simulink model "PistonController3"  (R2013a)
settings: Solver=FixedStepDiscrete  StartTime=0.0  StopTime=30  FixedStep=0.001  RelTol=1e-3
InitFcn:
  | % PI gains
  | 
  | K1_crit = 17.0;
  | T1_crit = 1.75;
  | K2_crit = K1_crit;
  | T2_crit = T1_crit;
  | K3_crit = K1_crit;
  | T3_crit = T1_crit;
  | K4_crit = K1_crit;
  | T4_crit = T1_crit;
  | K5_crit = 5.0;
  | T5_crit = 0.5;
  | K6_crit = 17.0;
  | T6_crit = 1.75;
  | KG_crit = 10.0;
  | TG_crit = 1.75;
  | 
  | 
  | P1 = 0.2*K1_crit;
  | I1 = 3.0*P1/T1_crit;
  | D1 = P1*T1_crit/3.0;
  | N1 = 10.0;
  | 
  | P2 = 0.2*K2_crit;
  | I2 = 3.0*P2/T2_crit;
  | D2 = P2*T2_crit/3.0;
  | N2 = 10.0;
  | 
  | P3 = 0.2*K3_crit;
  | I3 = 3.0*P3/T3_crit;
  | D3 = P3*T3_crit/3.0;
  | N3 = 10.0;
  | 
  | P4 = 0.2*K4_crit;
  | I4 = 3.0*P4/T4_crit;
  | D4 = P4*T4_crit/3.0;
  | N4 = 10.0;
  | 
  | P5 = 0.45*K5_crit;
  | I5 = 1.2*P5/T5_crit;
  | D5 = 0; %P5*T5_crit/3.0;
  | N5 = 10.0;
  | 
  | P6 = 0.2*K6_crit;
  | I6 = 3.0*P6/T6_crit;
  | D6 = P6*T6_crit/3.0;
  | N6 = 10.0;
  | 
  | PG = 0.2*KG_crit;
  | IG = 3.0*PG/TG_crit;
  | DG = PG*TG_crit/3.0;
  | NG = 10.0;
  | 
  | % offsets
  | offset = 1000;
  | offset_grip = 0;
  | 
  | %Max Cylinder Displacements = Left = positive
  | max_pos1 = 2800;
  | min_pos1 = -2800;
  | 
  | max_pos2 = 3000;
  | min_pos2 = -2700;
  | 
  | max_pos3 = 3000;
  | min_pos3 = -3000;
  | 
  | max_pos4 = 2800;
  | min_pos4 = -2900;
  | 
  | max_pos5 = 2900;
  | min_pos5 = -2600;
  | 
  | max_pos6 = 2800;
  | min_pos6 = -2800;
  | 
  | max_posG = 1500;
  | 
  | %Max Control Efforts
  | max1 = 5600;
  | min1 = -5600;
  | 
  | max2 = 5700;
  | min2 = -5700;
  | 
  | max3 = 6000;
  | min3 = -6000;
  | 
  | max4 = 5700;
  | min4 = -5700;
  | 
  | max5 = 5500;
  | min5 = -5500;
  | 
  | max6 = 5600;
  | min6 = -5600;
  | 
  | maxG = 3000;
  | minG = -3000;
undefined symbols (not defined in the file): rtwindemocb_modeswitch, Serial_Port, Standard_Devices
libraries: rtwinlib x14, simulink x7
Description:
  | Packet Input/Output
  | 
  | This model shows how to transfer data through UDP
  | communication protocol using binary encoding. The model sends data
  | within one computer, from one UDP port to another. You can modify the
  | model to communicate between two computers by splitting this model
  | into its send and receive parts and running the models on two computers.
  | The yellow blocks are used to send the data, the blue blocks
  | are used to receive the data. Then, please enter the IP addresses of the two
  | computers into the appropriate fields in the Board Setup dialog.
  | 
  | How to run this model in Normal Mode:
  | 
  | 1) Double-click the orange button to switch to Normal Mode if needed.
  | 2) Start the real-time execution using Simulation->Run.
  | 
  | How to run this model in External Mode:
  | 
  | 1) Double-click the orange button to switch to External Mode if needed.
  | 2) Build the model using Code->C/C++ Code->Build Model.
  | 3) Connect to the real-time code using Simulation->Connect To Target.
  | 4) Start the real-time execution using Simulation->Run.
settings Model: SimulationMode=external  ExtModeTrigDuration=30001  Creator=The MathWorks Inc.  LastModifiedBy=drl
settings DataIOCC: SignalLoggingSaveFormat=ModelDataLogs
settings OptimizationCC: InlineParams=on  InlineInvariantSignals=on  EnhancedBackFolding=on  ExpressionDepthLimit=2147483647  InitFltsAndDblsToZero=on  EfficientFloat2IntCast=on  EfficientMapNaN2IntZero=off  SimCompilerOptimization=On
settings DebuggingCC: MultiTaskDSMMsg=warning  MultiTaskCondExecSysMsg=none  FcnCallInpInsideContextMsg=EnableAllAsWarning  StrictBusMsg=None
settings HardwareCC: ProdIntDivRoundTo=Zero  ProdEndianess=LittleEndian  ProdHWDeviceType=32-bit Real-Time Windows Target  TargetIntDivRoundTo=Zero  TargetEndianess=LittleEndian  TargetHWDeviceType=32-bit Real-Time Windows Target
settings ModelReferenceCC: UpdateModelReferenceTargets=IfOutOfDate
settings SFSimCC: SFSimEcho=off
settings RTWCC: SystemTargetFile=rtwin.tlc  TemplateMakefile=rtwin.tmf  Description=Real-Time Windows Target  ProcessScript=rtwin_make_rtw_hook  IncludeERTFirstTime=on  RTWCompilerOptimization=On
settings RTWinTargetCC: TargetLibSuffix=_rtwin.lib  TargetPreCompLibLocation=C:\Program Files\MATLAB\R2013a\toolbox\rtw\targets\rtwin\lib\win64  CodeReplacementLibrary=ANSI_C  RTWinDir=C:/PROGRA~1/MATLAB/R2013a/toolbox/rtw/targets/rtwin  TargetArch=win64

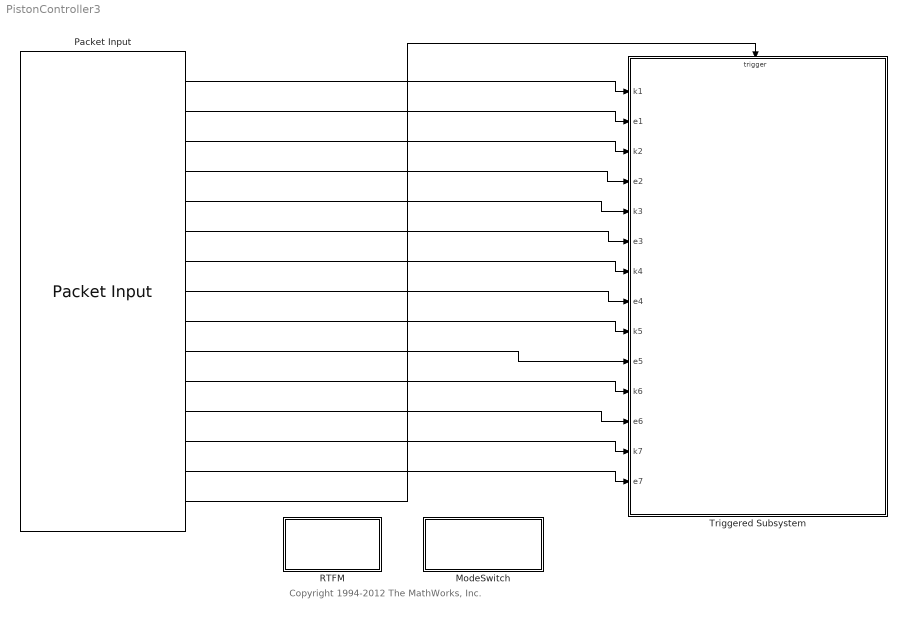
== system PistonController3 ==
  note: Copyright 1994-2012 The MathWorks, Inc.
  ModeSwitch : Subsystem  InitFcn=rtwindemocb_modeswitch('CheckKernel');  mask(Real-Time Windows Target Example Mode Switch){}
      settings: OpenFcn=rtwindemocb_modeswitch(gcbh);
      mask Display: disp('Switch To\nNormal Mode');
  Packet Input : rtwinlib/Packet Input  SampleTime=0.001  MaxMissedTicks=10000  ShowMissedTicks=off  YieldWhenWaiting=off  DrvName=Standard_Devices/Serial_Port  DrvAddress=39  DrvOptions=[57600 8 0 0 0 0 0 0]  PacketSize=14  DataTypes={'int8','int8','int8','int8','int8','int8','int8','int8','int8','int8','int8','int8','int8','int8'}  ShowReady=on  ShowError=off  PacketID=1  ByteOrder=1  ShowTimestamp=off
      settings: AttributesFormatString=Standard Devices\nSerial Port [27h]
  "RTFM " : Subsystem  mask(Real-Time Windows Target Example Info){}
      settings: OpenFcn=web(fullfile(fileparts(which(gcs)), 'html', [gcs '.html']), '-helpbrowser');
      mask Display: disp('Info')
  Triggered Subsystem : Subsystem  TreatAsAtomicUnit=on
  wires:
  Packet Input/10 -> Triggered Subsystem/10(e5)
  Packet Input/4 -> Triggered Subsystem/4(e2)
  Packet Input/12 -> Triggered Subsystem/12(e6)
  Packet Input/8 -> Triggered Subsystem/8(e4)
  Packet Input/9 -> Triggered Subsystem/9(k5)
  Packet Input/11 -> Triggered Subsystem/11(k6)
  Packet Input/5 -> Triggered Subsystem/5(k3)
  Packet Input/7 -> Triggered Subsystem/7(k4)
  Packet Input/6 -> Triggered Subsystem/6(e3)
  Packet Input/1 -> Triggered Subsystem/1(k1)
  Packet Input/3 -> Triggered Subsystem/3(k2)
  Packet Input/2 -> Triggered Subsystem/2(e1)
  Packet Input/13 -> Triggered Subsystem/13(k7)
  Packet Input/14 -> Triggered Subsystem/14(e7)
  Packet Input/15 -> Triggered Subsystem/Trigger

== system PistonController3/ModeSwitch ==

== system PistonController3/RTFM  ==

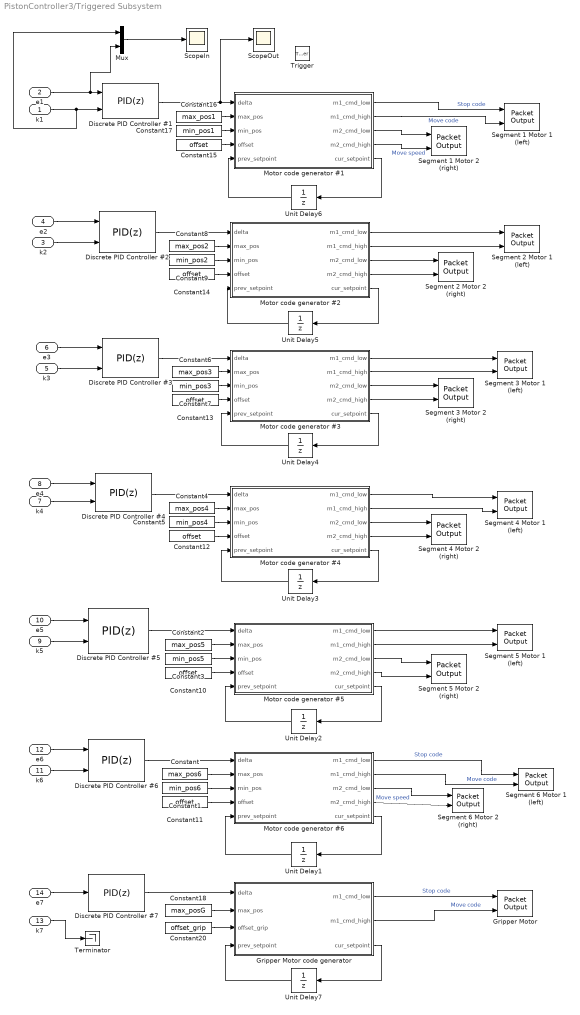
== system PistonController3/Triggered Subsystem ==
  k1 : Inport
  e1 : Inport  Port=2
  k2 : Inport  Port=3
  e2 : Inport  Port=4
  k3 : Inport  Port=5
  e3 : Inport  Port=6
  k4 : Inport  Port=7
  e4 : Inport  Port=8
  k5 : Inport  Port=9
  e5 : Inport  Port=10
  k6 : Inport  Port=11
  e6 : Inport  Port=12
  k7 : Inport  Port=13
  e7 : Inport  Port=14
  Trigger : TriggerPort
  Constant : Constant  Value=max_pos6
  Constant1 : Constant  Value=min_pos6
  Constant{10..15} (6 alike) : Constant  Value=offset
  Constant16 : Constant  Value=max_pos1
  Constant17 : Constant  Value=min_pos1
  Constant18 : Constant  Value=max_posG
  Constant2 : Constant  Value=max_pos5
  Constant20 : Constant  Value=offset_grip
  Constant3 : Constant  Value=min_pos5
  Constant4 : Constant  Value=max_pos4
  Constant5 : Constant  Value=min_pos4
  Constant6 : Constant  Value=max_pos3
  Constant7 : Constant  Value=min_pos3
  Constant8 : Constant  Value=max_pos2
  Constant9 : Constant  Value=min_pos2
  Discrete PID Controller #1 : simulink/Continuous/PID Controller  Controller=PID  TimeDomain=Discrete-time  SampleTime=-1  IntegratorMethod=Forward Euler  FilterMethod=Forward Euler  Form=Parallel  P=P1  I=I1  D=D1  N=N1  InitialConditionSource=internal  InitialConditionForIntegrator=0  InitialConditionForFilter=0  ExternalReset=either  LimitOutput=on  UpperSaturationLimit=max1  LowerSaturationLimit=min1  LinearizeAsGain=off  AntiWindupMode=clamping  Kb=1  TrackingMode=off  Kt=10  RndMeth=Nearest  SaturateOnIntegerOverflow=on  PParamMin=[]  PParamMax=[]  PParamDataTypeStr=double  IParamMin=[]  IParamMax=[]  IParamDataTypeStr=double  DParamMin=[]  DParamMax=[]  DParamDataTypeStr=double  NParamMin=[]  NParamMax=[]  NParamDataTypeStr=double  KbParamMin=[]  KbParamMax=[]  KtParamMin=[]  KtParamMax=[]  KtParamDataTypeStr=double  POutMin=[]  POutMax=[]  POutDataTypeStr=double  IOutMin=[]  IOutMax=[]  IOutDataTypeStr=double  DOutMin=[]  DOutMax=[]  DOutDataTypeStr=double  NOutMin=[]  NOutMax=[]  NOutDataTypeStr=double  KbOutMin=[]  KbOutMax=[]  KtOutMin=[]  KtOutMax=[]  KtOutDataTypeStr=double  IntegratorOutMin=[]  IntegratorOutMax=[]  IntegratorOutDataTypeStr=double  FilterOutMin=[]  FilterOutMax=[]  FilterOutDataTypeStr=double  SumOutMin=[]  SumOutMax=[]  SumOutDataTypeStr=double  SumI1OutMin=[]  SumI1OutMax=[]  SumI1OutDataTypeStr=double  SumI2OutMin=[]  SumI2OutMax=[]  SumI3OutMin=[]  SumI3OutMax=[]  SumI3OutDataTypeStr=double  SumDOutMin=[]  SumDOutMax=[]  SumDOutDataTypeStr=double  SumAccumDataTypeStr=double  SumI1AccumDataTypeStr=double  SumI3AccumDataTypeStr=double  SumDAccumDataTypeStr=double  SaturationOutMin=[]  SaturationOutMax=[]  SaturationOutDataTypeStr=double  IntegratorContinuousStateAttributes=''  IntegratorStateMustResolveToSignalObject=off  IntegratorRTWStateStorageClass=Auto  FilterContinuousStateAttributes=''  FilterStateMustResolveToSignalObject=off  FilterRTWStateStorageClass=Auto
  Discrete PID Controller #2 : simulink/Continuous/PID Controller  Controller=PID  TimeDomain=Discrete-time  SampleTime=-1  IntegratorMethod=Forward Euler  FilterMethod=Forward Euler  Form=Parallel  P=P2  I=I2  D=D2  N=N2  InitialConditionSource=internal  InitialConditionForIntegrator=0  InitialConditionForFilter=0  ExternalReset=either  LimitOutput=on  UpperSaturationLimit=max2  LowerSaturationLimit=min2  LinearizeAsGain=off  AntiWindupMode=clamping  Kb=1  TrackingMode=off  Kt=10  RndMeth=Nearest  SaturateOnIntegerOverflow=on  PParamMin=[]  PParamMax=[]  PParamDataTypeStr=double  IParamMin=[]  IParamMax=[]  IParamDataTypeStr=double  DParamMin=[]  DParamMax=[]  DParamDataTypeStr=double  NParamMin=[]  NParamMax=[]  NParamDataTypeStr=double  KbParamMin=[]  KbParamMax=[]  KtParamMin=[]  KtParamMax=[]  KtParamDataTypeStr=double  POutMin=[]  POutMax=[]  POutDataTypeStr=double  IOutMin=[]  IOutMax=[]  IOutDataTypeStr=double  DOutMin=[]  DOutMax=[]  DOutDataTypeStr=double  NOutMin=[]  NOutMax=[]  NOutDataTypeStr=double  KbOutMin=[]  KbOutMax=[]  KtOutMin=[]  KtOutMax=[]  KtOutDataTypeStr=double  IntegratorOutMin=[]  IntegratorOutMax=[]  IntegratorOutDataTypeStr=double  FilterOutMin=[]  FilterOutMax=[]  FilterOutDataTypeStr=double  SumOutMin=[]  SumOutMax=[]  SumOutDataTypeStr=double  SumI1OutMin=[]  SumI1OutMax=[]  SumI1OutDataTypeStr=double  SumI2OutMin=[]  SumI2OutMax=[]  SumI3OutMin=[]  SumI3OutMax=[]  SumI3OutDataTypeStr=double  SumDOutMin=[]  SumDOutMax=[]  SumDOutDataTypeStr=double  SumAccumDataTypeStr=double  SumI1AccumDataTypeStr=double  SumI3AccumDataTypeStr=double  SumDAccumDataTypeStr=double  SaturationOutMin=[]  SaturationOutMax=[]  SaturationOutDataTypeStr=double  IntegratorContinuousStateAttributes=''  IntegratorStateMustResolveToSignalObject=off  IntegratorRTWStateStorageClass=Auto  FilterContinuousStateAttributes=''  FilterStateMustResolveToSignalObject=off  FilterRTWStateStorageClass=Auto
  Discrete PID Controller #3 : simulink/Continuous/PID Controller  Controller=PID  TimeDomain=Discrete-time  SampleTime=-1  IntegratorMethod=Forward Euler  FilterMethod=Forward Euler  Form=Parallel  P=P3  I=I3  D=D3  N=N3  InitialConditionSource=internal  InitialConditionForIntegrator=0  InitialConditionForFilter=0  ExternalReset=either  LimitOutput=on  UpperSaturationLimit=max3  LowerSaturationLimit=min3  LinearizeAsGain=off  AntiWindupMode=clamping  Kb=1  TrackingMode=off  Kt=10  RndMeth=Nearest  SaturateOnIntegerOverflow=on  PParamMin=[]  PParamMax=[]  PParamDataTypeStr=double  IParamMin=[]  IParamMax=[]  IParamDataTypeStr=double  DParamMin=[]  DParamMax=[]  DParamDataTypeStr=double  NParamMin=[]  NParamMax=[]  NParamDataTypeStr=double  KbParamMin=[]  KbParamMax=[]  KtParamMin=[]  KtParamMax=[]  KtParamDataTypeStr=double  POutMin=[]  POutMax=[]  POutDataTypeStr=double  IOutMin=[]  IOutMax=[]  IOutDataTypeStr=double  DOutMin=[]  DOutMax=[]  DOutDataTypeStr=double  NOutMin=[]  NOutMax=[]  NOutDataTypeStr=double  KbOutMin=[]  KbOutMax=[]  KtOutMin=[]  KtOutMax=[]  KtOutDataTypeStr=double  IntegratorOutMin=[]  IntegratorOutMax=[]  IntegratorOutDataTypeStr=double  FilterOutMin=[]  FilterOutMax=[]  FilterOutDataTypeStr=double  SumOutMin=[]  SumOutMax=[]  SumOutDataTypeStr=double  SumI1OutMin=[]  SumI1OutMax=[]  SumI1OutDataTypeStr=double  SumI2OutMin=[]  SumI2OutMax=[]  SumI3OutMin=[]  SumI3OutMax=[]  SumI3OutDataTypeStr=double  SumDOutMin=[]  SumDOutMax=[]  SumDOutDataTypeStr=double  SumAccumDataTypeStr=double  SumI1AccumDataTypeStr=double  SumI3AccumDataTypeStr=double  SumDAccumDataTypeStr=double  SaturationOutMin=[]  SaturationOutMax=[]  SaturationOutDataTypeStr=double  IntegratorContinuousStateAttributes=''  IntegratorStateMustResolveToSignalObject=off  IntegratorRTWStateStorageClass=Auto  FilterContinuousStateAttributes=''  FilterStateMustResolveToSignalObject=off  FilterRTWStateStorageClass=Auto
  Discrete PID Controller #4 : simulink/Continuous/PID Controller  Controller=PID  TimeDomain=Discrete-time  SampleTime=-1  IntegratorMethod=Forward Euler  FilterMethod=Forward Euler  Form=Parallel  P=P4  I=I4  D=D4  N=N4  InitialConditionSource=internal  InitialConditionForIntegrator=0  InitialConditionForFilter=0  ExternalReset=either  LimitOutput=on  UpperSaturationLimit=max4  LowerSaturationLimit=min4  LinearizeAsGain=off  AntiWindupMode=clamping  Kb=1  TrackingMode=off  Kt=10  RndMeth=Nearest  SaturateOnIntegerOverflow=on  PParamMin=[]  PParamMax=[]  PParamDataTypeStr=double  IParamMin=[]  IParamMax=[]  IParamDataTypeStr=double  DParamMin=[]  DParamMax=[]  DParamDataTypeStr=double  NParamMin=[]  NParamMax=[]  NParamDataTypeStr=double  KbParamMin=[]  KbParamMax=[]  KtParamMin=[]  KtParamMax=[]  KtParamDataTypeStr=double  POutMin=[]  POutMax=[]  POutDataTypeStr=double  IOutMin=[]  IOutMax=[]  IOutDataTypeStr=double  DOutMin=[]  DOutMax=[]  DOutDataTypeStr=double  NOutMin=[]  NOutMax=[]  NOutDataTypeStr=double  KbOutMin=[]  KbOutMax=[]  KtOutMin=[]  KtOutMax=[]  KtOutDataTypeStr=double  IntegratorOutMin=[]  IntegratorOutMax=[]  IntegratorOutDataTypeStr=double  FilterOutMin=[]  FilterOutMax=[]  FilterOutDataTypeStr=double  SumOutMin=[]  SumOutMax=[]  SumOutDataTypeStr=double  SumI1OutMin=[]  SumI1OutMax=[]  SumI1OutDataTypeStr=double  SumI2OutMin=[]  SumI2OutMax=[]  SumI3OutMin=[]  SumI3OutMax=[]  SumI3OutDataTypeStr=double  SumDOutMin=[]  SumDOutMax=[]  SumDOutDataTypeStr=double  SumAccumDataTypeStr=double  SumI1AccumDataTypeStr=double  SumI3AccumDataTypeStr=double  SumDAccumDataTypeStr=double  SaturationOutMin=[]  SaturationOutMax=[]  SaturationOutDataTypeStr=double  IntegratorContinuousStateAttributes=''  IntegratorStateMustResolveToSignalObject=off  IntegratorRTWStateStorageClass=Auto  FilterContinuousStateAttributes=''  FilterStateMustResolveToSignalObject=off  FilterRTWStateStorageClass=Auto
  Discrete PID Controller #5 : simulink/Continuous/PID Controller  Controller=PID  TimeDomain=Discrete-time  SampleTime=-1  IntegratorMethod=Forward Euler  FilterMethod=Forward Euler  Form=Parallel  P=P5  I=I5  D=D5  N=N5  InitialConditionSource=internal  InitialConditionForIntegrator=0  InitialConditionForFilter=0  ExternalReset=either  LimitOutput=on  UpperSaturationLimit=max5  LowerSaturationLimit=min5  LinearizeAsGain=off  AntiWindupMode=clamping  Kb=1  TrackingMode=off  Kt=10  RndMeth=Nearest  SaturateOnIntegerOverflow=on  PParamMin=[]  PParamMax=[]  PParamDataTypeStr=double  IParamMin=[]  IParamMax=[]  IParamDataTypeStr=double  DParamMin=[]  DParamMax=[]  DParamDataTypeStr=double  NParamMin=[]  NParamMax=[]  NParamDataTypeStr=double  KbParamMin=[]  KbParamMax=[]  KtParamMin=[]  KtParamMax=[]  KtParamDataTypeStr=double  POutMin=[]  POutMax=[]  POutDataTypeStr=double  IOutMin=[]  IOutMax=[]  IOutDataTypeStr=double  DOutMin=[]  DOutMax=[]  DOutDataTypeStr=double  NOutMin=[]  NOutMax=[]  NOutDataTypeStr=double  KbOutMin=[]  KbOutMax=[]  KtOutMin=[]  KtOutMax=[]  KtOutDataTypeStr=double  IntegratorOutMin=[]  IntegratorOutMax=[]  IntegratorOutDataTypeStr=double  FilterOutMin=[]  FilterOutMax=[]  FilterOutDataTypeStr=double  SumOutMin=[]  SumOutMax=[]  SumOutDataTypeStr=double  SumI1OutMin=[]  SumI1OutMax=[]  SumI1OutDataTypeStr=double  SumI2OutMin=[]  SumI2OutMax=[]  SumI3OutMin=[]  SumI3OutMax=[]  SumI3OutDataTypeStr=double  SumDOutMin=[]  SumDOutMax=[]  SumDOutDataTypeStr=double  SumAccumDataTypeStr=double  SumI1AccumDataTypeStr=double  SumI3AccumDataTypeStr=double  SumDAccumDataTypeStr=double  SaturationOutMin=[]  SaturationOutMax=[]  SaturationOutDataTypeStr=double  IntegratorContinuousStateAttributes=''  IntegratorStateMustResolveToSignalObject=off  IntegratorRTWStateStorageClass=Auto  FilterContinuousStateAttributes=''  FilterStateMustResolveToSignalObject=off  FilterRTWStateStorageClass=Auto
  Discrete PID Controller #6 : simulink/Continuous/PID Controller  Controller=PID  TimeDomain=Discrete-time  SampleTime=-1  IntegratorMethod=Forward Euler  FilterMethod=Forward Euler  Form=Parallel  P=P6  I=I6  D=D6  N=N6  InitialConditionSource=internal  InitialConditionForIntegrator=0  InitialConditionForFilter=0  ExternalReset=either  LimitOutput=on  UpperSaturationLimit=max6  LowerSaturationLimit=min6  LinearizeAsGain=off  AntiWindupMode=clamping  Kb=1  TrackingMode=off  Kt=10  RndMeth=Nearest  SaturateOnIntegerOverflow=on  PParamMin=[]  PParamMax=[]  PParamDataTypeStr=double  IParamMin=[]  IParamMax=[]  IParamDataTypeStr=double  DParamMin=[]  DParamMax=[]  DParamDataTypeStr=double  NParamMin=[]  NParamMax=[]  NParamDataTypeStr=double  KbParamMin=[]  KbParamMax=[]  KtParamMin=[]  KtParamMax=[]  KtParamDataTypeStr=double  POutMin=[]  POutMax=[]  POutDataTypeStr=double  IOutMin=[]  IOutMax=[]  IOutDataTypeStr=double  DOutMin=[]  DOutMax=[]  DOutDataTypeStr=double  NOutMin=[]  NOutMax=[]  NOutDataTypeStr=double  KbOutMin=[]  KbOutMax=[]  KtOutMin=[]  KtOutMax=[]  KtOutDataTypeStr=double  IntegratorOutMin=[]  IntegratorOutMax=[]  IntegratorOutDataTypeStr=double  FilterOutMin=[]  FilterOutMax=[]  FilterOutDataTypeStr=double  SumOutMin=[]  SumOutMax=[]  SumOutDataTypeStr=double  SumI1OutMin=[]  SumI1OutMax=[]  SumI1OutDataTypeStr=double  SumI2OutMin=[]  SumI2OutMax=[]  SumI3OutMin=[]  SumI3OutMax=[]  SumI3OutDataTypeStr=double  SumDOutMin=[]  SumDOutMax=[]  SumDOutDataTypeStr=double  SumAccumDataTypeStr=double  SumI1AccumDataTypeStr=double  SumI3AccumDataTypeStr=double  SumDAccumDataTypeStr=double  SaturationOutMin=[]  SaturationOutMax=[]  SaturationOutDataTypeStr=double  IntegratorContinuousStateAttributes=''  IntegratorStateMustResolveToSignalObject=off  IntegratorRTWStateStorageClass=Auto  FilterContinuousStateAttributes=''  FilterStateMustResolveToSignalObject=off  FilterRTWStateStorageClass=Auto
  Discrete PID Controller #7 : simulink/Continuous/PID Controller  Controller=PID  TimeDomain=Discrete-time  SampleTime=-1  IntegratorMethod=Forward Euler  FilterMethod=Forward Euler  Form=Parallel  P=PG  I=IG  D=DG  N=NG  InitialConditionSource=internal  InitialConditionForIntegrator=0  InitialConditionForFilter=0  ExternalReset=none  LimitOutput=on  UpperSaturationLimit=maxG  LowerSaturationLimit=minG  LinearizeAsGain=off  AntiWindupMode=clamping  Kb=1  TrackingMode=off  Kt=10  RndMeth=Nearest  SaturateOnIntegerOverflow=on  PParamMin=[]  PParamMax=[]  PParamDataTypeStr=double  IParamMin=[]  IParamMax=[]  IParamDataTypeStr=double  DParamMin=[]  DParamMax=[]  DParamDataTypeStr=double  NParamMin=[]  NParamMax=[]  NParamDataTypeStr=double  KbParamMin=[]  KbParamMax=[]  KtParamMin=[]  KtParamMax=[]  KtParamDataTypeStr=double  POutMin=[]  POutMax=[]  POutDataTypeStr=double  IOutMin=[]  IOutMax=[]  IOutDataTypeStr=double  DOutMin=[]  DOutMax=[]  DOutDataTypeStr=double  NOutMin=[]  NOutMax=[]  NOutDataTypeStr=double  KbOutMin=[]  KbOutMax=[]  KtOutMin=[]  KtOutMax=[]  KtOutDataTypeStr=double  IntegratorOutMin=[]  IntegratorOutMax=[]  IntegratorOutDataTypeStr=double  FilterOutMin=[]  FilterOutMax=[]  FilterOutDataTypeStr=double  SumOutMin=[]  SumOutMax=[]  SumOutDataTypeStr=double  SumI1OutMin=[]  SumI1OutMax=[]  SumI1OutDataTypeStr=double  SumI2OutMin=[]  SumI2OutMax=[]  SumI3OutMin=[]  SumI3OutMax=[]  SumI3OutDataTypeStr=double  SumDOutMin=[]  SumDOutMax=[]  SumDOutDataTypeStr=double  SumAccumDataTypeStr=double  SumI1AccumDataTypeStr=double  SumI3AccumDataTypeStr=double  SumDAccumDataTypeStr=double  SaturationOutMin=[]  SaturationOutMax=[]  SaturationOutDataTypeStr=double  IntegratorContinuousStateAttributes=''  IntegratorStateMustResolveToSignalObject=off  IntegratorRTWStateStorageClass=Auto  FilterContinuousStateAttributes=''  FilterStateMustResolveToSignalObject=off  FilterRTWStateStorageClass=Auto
  Gripper Motor : rtwinlib/Packet Output  SampleTime=-1  MaxMissedTicks=10  ShowMissedTicks=off  YieldWhenWaiting=off  DrvName=Standard_Devices/Serial_Port  DrvAddress=68  DrvOptions=[57600 8 0 0 0 0 0 0]  PacketSize=2  DataTypes={'uint8','uint8'}  ShowReady=off  ShowError=off  PacketID=1  ByteOrder=1  InitialValue=[192, 0]  FinalValue=[192, 0]
      settings: AttributesFormatString=Standard Devices\nSerial Port [44h]
  "Gripper Motor code generator " : MATLAB Function  TreatAsAtomicUnit=on
  Motor code generator #1 : MATLAB Function  TreatAsAtomicUnit=on
  Motor code generator #2 : MATLAB Function  TreatAsAtomicUnit=on
  Motor code generator #3 : MATLAB Function  TreatAsAtomicUnit=on
  Motor code generator #4 : MATLAB Function  TreatAsAtomicUnit=on
  Motor code generator #5 : MATLAB Function  TreatAsAtomicUnit=on
  Motor code generator #6 : MATLAB Function  TreatAsAtomicUnit=on
  Mux : Mux  Inputs=2
  ScopeIn : Scope
      settings: ShowLegends=on  YMin=-35  YMax=35  SaveName=Scopelnput  MaxDataPoints=30000
  ScopeOut : Scope
      settings: ShowLegends=on  YMin=-35  YMax=35  SaveName=ScopeControlEffort  MaxDataPoints=30000
  Segment 1 Motor 1 (left) : rtwinlib/Packet Output  SampleTime=-1  MaxMissedTicks=10  ShowMissedTicks=off  YieldWhenWaiting=off  DrvName=Standard_Devices/Serial_Port  DrvAddress=19  DrvOptions=[57600 8 0 0 0 0 0 0]  PacketSize=2  DataTypes={'uint8','uint8'}  ShowReady=off  ShowError=off  PacketID=1  ByteOrder=1  InitialValue=[200, 31]  FinalValue=[200, 31]
      settings: AttributesFormatString=Standard Devices\nSerial Port [13h]
  Segment 1 Motor 2 (right) : rtwinlib/Packet Output  SampleTime=-1  MaxMissedTicks=10  ShowMissedTicks=off  YieldWhenWaiting=off  DrvName=Standard_Devices/Serial_Port  DrvAddress=22  DrvOptions=[57600 8 0 0 0 0 0 0]  PacketSize=2  DataTypes={'uint8','uint8'}  ShowReady=off  ShowError=off  PacketID=1  ByteOrder=1  InitialValue=[200, 31]  FinalValue=[200, 31]
      settings: AttributesFormatString=Standard Devices\nSerial Port [16h]
  Segment 2 Motor 1 (left) : rtwinlib/Packet Output  SampleTime=-1  MaxMissedTicks=10  ShowMissedTicks=off  YieldWhenWaiting=off  DrvName=Standard_Devices/Serial_Port  DrvAddress=23  DrvOptions=[57600 8 0 0 0 0 0 0]  PacketSize=2  DataTypes={'uint8','uint8'}  ShowReady=off  ShowError=off  PacketID=1  ByteOrder=1  InitialValue=[200, 31]  FinalValue=[200, 31]
      settings: AttributesFormatString=Standard Devices\nSerial Port [17h]
  Segment 2 Motor 2 (right) : rtwinlib/Packet Output  SampleTime=-1  MaxMissedTicks=10  ShowMissedTicks=off  YieldWhenWaiting=off  DrvName=Standard_Devices/Serial_Port  DrvAddress=25  DrvOptions=[57600 8 0 0 0 0 0 0]  PacketSize=2  DataTypes={'uint8','uint8'}  ShowReady=off  ShowError=off  PacketID=1  ByteOrder=1  InitialValue=[200, 31]  FinalValue=[200, 31]
      settings: AttributesFormatString=Standard Devices\nSerial Port [19h]
  Segment 3 Motor 1 (left) : rtwinlib/Packet Output  SampleTime=-1  MaxMissedTicks=10  ShowMissedTicks=off  YieldWhenWaiting=off  DrvName=Standard_Devices/Serial_Port  DrvAddress=17  DrvOptions=[57600 8 0 0 0 0 0 0]  PacketSize=2  DataTypes={'uint8','uint8'}  ShowReady=off  ShowError=off  PacketID=1  ByteOrder=1  InitialValue=[200, 31]  FinalValue=[200, 31]
      settings: AttributesFormatString=Standard Devices\nSerial Port [11h]
  Segment 3 Motor 2 (right) : rtwinlib/Packet Output  SampleTime=-1  MaxMissedTicks=10  ShowMissedTicks=off  YieldWhenWaiting=off  DrvName=Standard_Devices/Serial_Port  DrvAddress=16  DrvOptions=[57600 8 0 0 0 0 0 0]  PacketSize=2  DataTypes={'uint8','uint8'}  ShowReady=off  ShowError=off  PacketID=1  ByteOrder=1  InitialValue=[200, 31]  FinalValue=[200, 31]
      settings: AttributesFormatString=Standard Devices\nSerial Port [10h]
  Segment 4 Motor 1 (left) : rtwinlib/Packet Output  SampleTime=-1  MaxMissedTicks=10  ShowMissedTicks=off  YieldWhenWaiting=off  DrvName=Standard_Devices/Serial_Port  DrvAddress=27  DrvOptions=[57600 8 0 0 0 0 0 0]  PacketSize=2  DataTypes={'uint8','uint8'}  ShowReady=off  ShowError=off  PacketID=1  ByteOrder=1  InitialValue=[200, 31]  FinalValue=[200, 31]
      settings: AttributesFormatString=Standard Devices\nSerial Port [1Bh]
  Segment 4 Motor 2 (right) : rtwinlib/Packet Output  SampleTime=-1  MaxMissedTicks=10  ShowMissedTicks=off  YieldWhenWaiting=off  DrvName=Standard_Devices/Serial_Port  DrvAddress=29  DrvOptions=[57600 8 0 0 0 0 0 0]  PacketSize=2  DataTypes={'uint8','uint8'}  ShowReady=off  ShowError=off  PacketID=1  ByteOrder=1  InitialValue=[200, 31]  FinalValue=[200, 31]
      settings: AttributesFormatString=Standard Devices\nSerial Port [1Dh]
  Segment 5 Motor 1 (left) : rtwinlib/Packet Output  SampleTime=-1  MaxMissedTicks=10  ShowMissedTicks=off  YieldWhenWaiting=off  DrvName=Standard_Devices/Serial_Port  DrvAddress=31  DrvOptions=[57600 8 0 0 0 0 0 0]  PacketSize=2  DataTypes={'uint8','uint8'}  ShowReady=off  ShowError=off  PacketID=1  ByteOrder=1  InitialValue=[200, 31]  FinalValue=[200, 31]
      settings: AttributesFormatString=Standard Devices\nSerial Port [1Fh]
  Segment 5 Motor 2 (right) : rtwinlib/Packet Output  SampleTime=-1  MaxMissedTicks=10  ShowMissedTicks=off  YieldWhenWaiting=off  DrvName=Standard_Devices/Serial_Port  DrvAddress=34  DrvOptions=[57600 8 0 0 0 0 0 0]  PacketSize=2  DataTypes={'uint8','uint8'}  ShowReady=off  ShowError=off  PacketID=1  ByteOrder=1  InitialValue=[200, 31]  FinalValue=[200, 31]
      settings: AttributesFormatString=Standard Devices\nSerial Port [22h]
  Segment 6 Motor 1 (left) : rtwinlib/Packet Output  SampleTime=-1  MaxMissedTicks=10  ShowMissedTicks=off  YieldWhenWaiting=off  DrvName=Standard_Devices/Serial_Port  DrvAddress=35  DrvOptions=[57600 8 0 0 0 0 0 0]  PacketSize=2  DataTypes={'uint8','uint8'}  ShowReady=off  ShowError=off  PacketID=1  ByteOrder=1  InitialValue=[200, 31]  FinalValue=[200, 31]
      settings: AttributesFormatString=Standard Devices\nSerial Port [23h]
  Segment 6 Motor 2 (right) : rtwinlib/Packet Output  SampleTime=-1  MaxMissedTicks=10  ShowMissedTicks=off  YieldWhenWaiting=off  DrvName=Standard_Devices/Serial_Port  DrvAddress=38  DrvOptions=[57600 8 0 0 0 0 0 0]  PacketSize=2  DataTypes={'uint8','uint8'}  ShowReady=off  ShowError=off  PacketID=1  ByteOrder=1  InitialValue=[200, 31]  FinalValue=[200, 31]
      settings: AttributesFormatString=Standard Devices\nSerial Port [26h]
  Terminator : Terminator
  Unit Delay{1..7} (7 alike) : UnitDelay  SampleTime=-1
  wires:
  e3/1 -> Discrete PID Controller #3/1
  Discrete PID Controller #3/1 -> Motor code generator #3/1(delta)
  k3/1 -> Discrete PID Controller #3/2
  Motor code generator #3/1(m1_cmd_low) -> Segment 3 Motor 1 (left)/1
  Motor code generator #3/2(m1_cmd_high) -> Segment 3 Motor 1 (left)/2
  Motor code generator #3/3(m2_cmd_low) -> Segment 3 Motor 2 (right)/1
  Discrete PID Controller #1/1 -> ScopeOut/1, Motor code generator #1/1(delta)
  k1/1 -> Discrete PID Controller #1/2, Mux/1
  Motor code generator #1/1(m1_cmd_low) -> Segment 1 Motor 1 (left)/1  "Stop code"
  Motor code generator #1/2(m1_cmd_high) -> Segment 1 Motor 1 (left)/2  "Move code"
  Motor code generator #1/3(m2_cmd_low) -> Segment 1 Motor 2 (right)/1
  Motor code generator #1/4(m2_cmd_high) -> Segment 1 Motor 2 (right)/2  "Move speed"
  e1/1 -> Discrete PID Controller #1/1, Mux/2
  Discrete PID Controller #2/1 -> Motor code generator #2/1(delta)
  k2/1 -> Discrete PID Controller #2/2
  Motor code generator #2/1(m1_cmd_low) -> Segment 2 Motor 1 (left)/1
  Motor code generator #2/2(m1_cmd_high) -> Segment 2 Motor 1 (left)/2
  Motor code generator #2/3(m2_cmd_low) -> Segment 2 Motor 2 (right)/1
  Motor code generator #2/4(m2_cmd_high) -> Segment 2 Motor 2 (right)/2
  e2/1 -> Discrete PID Controller #2/1
  Discrete PID Controller #4/1 -> Motor code generator #4/1(delta)
  Motor code generator #4/1(m1_cmd_low) -> Segment 4 Motor 1 (left)/1
  Motor code generator #4/2(m1_cmd_high) -> Segment 4 Motor 1 (left)/2
  Motor code generator #4/3(m2_cmd_low) -> Segment 4 Motor 2 (right)/1
  Motor code generator #4/4(m2_cmd_high) -> Segment 4 Motor 2 (right)/2
  e4/1 -> Discrete PID Controller #4/1
  Motor code generator #5/4(m2_cmd_high) -> Segment 5 Motor 2 (right)/2
  e6/1 -> Discrete PID Controller #6/1
  Discrete PID Controller #6/1 -> Motor code generator #6/1(delta)
  Motor code generator #6/1(m1_cmd_low) -> Segment 6 Motor 1 (left)/1  "Stop code"
  Motor code generator #6/2(m1_cmd_high) -> Segment 6 Motor 1 (left)/2  "Move code"
  Motor code generator #6/3(m2_cmd_low) -> Segment 6 Motor 2 (right)/1
  Motor code generator #6/4(m2_cmd_high) -> Segment 6 Motor 2 (right)/2  "Move speed"
  e7/1 -> Discrete PID Controller #7/1
  "Gripper Motor code generator "/1(m1_cmd_low) -> Gripper Motor/1  "Stop code"
  "Gripper Motor code generator "/2(m1_cmd_high) -> Gripper Motor/2  "Move code"
  Mux/1 -> ScopeIn/1
  Motor code generator #6/5(cur_setpoint) -> Unit Delay1/1
  e5/1 -> Discrete PID Controller #5/1
  Constant/1 -> Motor code generator #6/2(max_pos)
  Constant1/1 -> Motor code generator #6/3(min_pos)
  Discrete PID Controller #5/1 -> Motor code generator #5/1(delta)
  Motor code generator #5/5(cur_setpoint) -> Unit Delay2/1
  Constant2/1 -> Motor code generator #5/2(max_pos)
  Constant3/1 -> Motor code generator #5/3(min_pos)
  Motor code generator #5/1(m1_cmd_low) -> Segment 5 Motor 1 (left)/1
  Motor code generator #5/2(m1_cmd_high) -> Segment 5 Motor 1 (left)/2
  Motor code generator #5/3(m2_cmd_low) -> Segment 5 Motor 2 (right)/1
  k4/1 -> Discrete PID Controller #4/2
  k6/1 -> Discrete PID Controller #6/2
  Motor code generator #4/5(cur_setpoint) -> Unit Delay3/1
  Constant4/1 -> Motor code generator #4/2(max_pos)
  Constant5/1 -> Motor code generator #4/3(min_pos)
  Constant7/1 -> Motor code generator #3/3(min_pos)
  Motor code generator #3/4(m2_cmd_high) -> Segment 3 Motor 2 (right)/2
  Motor code generator #3/5(cur_setpoint) -> Unit Delay4/1
  Constant6/1 -> Motor code generator #3/2(max_pos)
  Constant9/1 -> Motor code generator #2/3(min_pos)
  Motor code generator #2/5(cur_setpoint) -> Unit Delay5/1
  Constant8/1 -> Motor code generator #2/2(max_pos)
  Unit Delay2/1 -> Motor code generator #5/5(prev_setpoint)
  Constant10/1 -> Motor code generator #5/4(offset)
  Constant11/1 -> Motor code generator #6/4(offset)
  Unit Delay1/1 -> Motor code generator #6/5(prev_setpoint)
  Constant12/1 -> Motor code generator #4/4(offset)
  Unit Delay3/1 -> Motor code generator #4/5(prev_setpoint)
  Unit Delay6/1 -> Motor code generator #1/5(prev_setpoint)
  Motor code generator #1/5(cur_setpoint) -> Unit Delay6/1
  Constant15/1 -> Motor code generator #1/4(offset)
  Constant17/1 -> Motor code generator #1/3(min_pos)
  Constant16/1 -> Motor code generator #1/2(max_pos)
  Constant14/1 -> Motor code generator #2/4(offset)
  Unit Delay5/1 -> Motor code generator #2/5(prev_setpoint)
  Constant13/1 -> Motor code generator #3/4(offset)
  Discrete PID Controller #7/1 -> "Gripper Motor code generator "/1(delta)
  Constant18/1 -> "Gripper Motor code generator "/2(max_pos)
  Constant20/1 -> "Gripper Motor code generator "/3(offset_grip)
  "Gripper Motor code generator "/3(cur_setpoint) -> Unit Delay7/1
  Unit Delay7/1 -> "Gripper Motor code generator "/4(prev_setpoint)
  k7/1 -> Terminator/1
  Unit Delay4/1 -> Motor code generator #3/5(prev_setpoint)
  k5/1 -> Discrete PID Controller #5/2

== matlab function PistonController3/Triggered Subsystem/Motor code generator #1 ==
  data: m1_cmd_low output; delta input; m1_cmd_high output; m2_cmd_low output; max_pos input; m2_cmd_high output; min_pos input; offset input; prev_setpoint input; cur_setpoint output
function [m1_cmd_low, m1_cmd_high, m2_cmd_low, m2_cmd_high,cur_setpoint] = ...
    code_gen(delta,max_pos,min_pos,offset,prev_setpoint)

% New Conrol Effort
pos_setpoint =  prev_setpoint + delta;

% Check for Saturation
if (pos_setpoint >= max_pos)
	pos_setpoint = max_pos;
elseif (pos_setpoint <= min_pos)
    pos_setpoint = min_pos;
end
% Feedback setpoint for next time step
cur_setpoint = pos_setpoint;

% Translate to two pistons which both start with the same offset
if (pos_setpoint >= 0)
motor_2_cmd = uint16(pos_setpoint+offset);
motor_1_cmd = uint16(0 + offset);
else
motor_2_cmd = uint16(0+ offset);
motor_1_cmd  = uint16(abs(pos_setpoint)+offset);
end

%% Prepare motor output
m1_cmd_low = uint8(uint16(192) + bitand(motor_1_cmd, uint16(31)));
m1_cmd_high = uint8(bitand(bitshift(motor_1_cmd, -5), uint16(127)));

m2_cmd_low = uint8(uint16(192) + bitand(motor_2_cmd, uint16(31)));
m2_cmd_high = uint8(bitand(bitshift(motor_2_cmd, -5), uint16(127)));

== matlab function PistonController3/Triggered Subsystem/Motor code generator #2 ==
  data: m1_cmd_low output; m1_cmd_high output; m2_cmd_low output; delta input; max_pos input; min_pos input; m2_cmd_high output; offset input; cur_setpoint output; prev_setpoint input
function [m1_cmd_low, m1_cmd_high, m2_cmd_low, m2_cmd_high,cur_setpoint] = ...
    code_gen(delta,max_pos,min_pos,offset,prev_setpoint)

% New Conrol Effort
pos_setpoint =  prev_setpoint + delta;

% Check for Saturation
if (pos_setpoint >= max_pos)
	pos_setpoint = max_pos;
elseif (pos_setpoint <= min_pos)
    pos_setpoint = min_pos;
end
% Feedback setpoint for next time step
cur_setpoint = pos_setpoint;

% Translate to two pistons which both start with the same offset
if (pos_setpoint >= 0)
motor_2_cmd = uint16(pos_setpoint+offset);
motor_1_cmd = uint16(0 + offset);
else
motor_2_cmd = uint16(0+ offset);
motor_1_cmd  = uint16(abs(pos_setpoint)+offset);
end

%% Prepare motor output
m1_cmd_low = uint8(uint16(192) + bitand(motor_1_cmd, uint16(31)));
m1_cmd_high = uint8(bitand(bitshift(motor_1_cmd, -5), uint16(127)));

m2_cmd_low = uint8(uint16(192) + bitand(motor_2_cmd, uint16(31)));
m2_cmd_high = uint8(bitand(bitshift(motor_2_cmd, -5), uint16(127)));

== matlab function PistonController3/Triggered Subsystem/Motor code generator #4 ==
  data: m1_cmd_low output; m1_cmd_high output; m2_cmd_low output; delta input; max_pos input; min_pos input; m2_cmd_high output; offset input; cur_setpoint output; prev_setpoint input
function [m1_cmd_low, m1_cmd_high, m2_cmd_low, m2_cmd_high,cur_setpoint] = ...
    code_gen(delta,max_pos,min_pos,offset,prev_setpoint)

% New Conrol Effort
pos_setpoint =  prev_setpoint + delta;

% Check for Saturation
if (pos_setpoint >= max_pos)
	pos_setpoint = max_pos;
elseif (pos_setpoint <= min_pos)
    pos_setpoint = min_pos;
end
% Feedback setpoint for next time step
cur_setpoint = pos_setpoint;

% Translate to two pistons which both start with the same offset
if (pos_setpoint >= 0)
motor_2_cmd = uint16(pos_setpoint+offset);
motor_1_cmd = uint16(0 + offset);
else
motor_2_cmd = uint16(0+ offset);
motor_1_cmd  = uint16(abs(pos_setpoint)+offset);
end

%% Prepare motor output
m1_cmd_low = uint8(uint16(192) + bitand(motor_1_cmd, uint16(31)));
m1_cmd_high = uint8(bitand(bitshift(motor_1_cmd, -5), uint16(127)));

m2_cmd_low = uint8(uint16(192) + bitand(motor_2_cmd, uint16(31)));
m2_cmd_high = uint8(bitand(bitshift(motor_2_cmd, -5), uint16(127)));

== matlab function PistonController3/Triggered Subsystem/Motor code generator #3 ==
  data: m1_cmd_low output; m1_cmd_high output; m2_cmd_low output; delta input; max_pos input; min_pos input; m2_cmd_high output; offset input; cur_setpoint output; prev_setpoint input
function [m1_cmd_low, m1_cmd_high, m2_cmd_low, m2_cmd_high,cur_setpoint] = ...
    code_gen(delta,max_pos,min_pos,offset,prev_setpoint)

% New Conrol Effort
pos_setpoint =  prev_setpoint + delta;

% Check for Saturation
if (pos_setpoint >= max_pos)
	pos_setpoint = max_pos;
elseif (pos_setpoint <= min_pos)
    pos_setpoint = min_pos;
end
% Feedback setpoint for next time step
cur_setpoint = pos_setpoint;

% Translate to two pistons which both start with the same offset
if (pos_setpoint >= 0)
motor_2_cmd = uint16(pos_setpoint+offset);
motor_1_cmd = uint16(0 + offset);
else
motor_2_cmd = uint16(0+ offset);
motor_1_cmd  = uint16(abs(pos_setpoint)+offset);
end

%% Prepare motor output
m1_cmd_low = uint8(uint16(192) + bitand(motor_1_cmd, uint16(31)));
m1_cmd_high = uint8(bitand(bitshift(motor_1_cmd, -5), uint16(127)));

m2_cmd_low = uint8(uint16(192) + bitand(motor_2_cmd, uint16(31)));
m2_cmd_high = uint8(bitand(bitshift(motor_2_cmd, -5), uint16(127)));

== matlab function PistonController3/Triggered Subsystem/Motor code generator #5 ==
  data: m1_cmd_low output; m1_cmd_high output; m2_cmd_low output; delta input; max_pos input; min_pos input; m2_cmd_high output; offset input; cur_setpoint output; prev_setpoint input
function [m1_cmd_low, m1_cmd_high, m2_cmd_low, m2_cmd_high,cur_setpoint] = ...
    code_gen(delta,max_pos,min_pos,offset,prev_setpoint)

% New Conrol Effort
pos_setpoint =  prev_setpoint + delta;

% Check for Saturation
if (pos_setpoint >= max_pos)
	pos_setpoint = max_pos;
elseif (pos_setpoint <= min_pos)
    pos_setpoint = min_pos;
end
% Feedback setpoint for next time step
cur_setpoint = pos_setpoint;

% Translate to two pistons which both start with the same offset
if (pos_setpoint >= 0)
motor_2_cmd = uint16(pos_setpoint+offset);
motor_1_cmd = uint16(0 + offset);
else
motor_2_cmd = uint16(0+ offset);
motor_1_cmd  = uint16(abs(pos_setpoint)+offset);
end

%% Prepare motor output
m1_cmd_low = uint8(uint16(192) + bitand(motor_1_cmd, uint16(31)));
m1_cmd_high = uint8(bitand(bitshift(motor_1_cmd, -5), uint16(127)));

m2_cmd_low = uint8(uint16(192) + bitand(motor_2_cmd, uint16(31)));
m2_cmd_high = uint8(bitand(bitshift(motor_2_cmd, -5), uint16(127)));

== matlab function PistonController3/Triggered Subsystem/Motor code generator #6 ==
  data: m1_cmd_low output; m1_cmd_high output; m2_cmd_low output; delta input; max_pos input; min_pos input; m2_cmd_high output; offset input; cur_setpoint output; prev_setpoint input
function [m1_cmd_low, m1_cmd_high, m2_cmd_low, m2_cmd_high,cur_setpoint] = ...
    code_gen(delta,max_pos,min_pos,offset,prev_setpoint)

% New Conrol Effort
pos_setpoint =  prev_setpoint + delta;

% Check for Saturation
if (pos_setpoint >= max_pos)
	pos_setpoint = max_pos;
elseif (pos_setpoint <= min_pos)
    pos_setpoint = min_pos;
end
% Feedback setpoint for next time step
cur_setpoint = pos_setpoint;

% Translate to two pistons which both start with the same offset
if (pos_setpoint >= 0)
motor_2_cmd = uint16(pos_setpoint+offset);
motor_1_cmd = uint16(0 + offset);
else
motor_2_cmd = uint16(0+ offset);
motor_1_cmd  = uint16(abs(pos_setpoint)+offset);
end

%% Prepare motor output
m1_cmd_low = uint8(uint16(192) + bitand(motor_1_cmd, uint16(31)));
m1_cmd_high = uint8(bitand(bitshift(motor_1_cmd, -5), uint16(127)));

m2_cmd_low = uint8(uint16(192) + bitand(motor_2_cmd, uint16(31)));
m2_cmd_high = uint8(bitand(bitshift(motor_2_cmd, -5), uint16(127)));

== matlab function PistonController3/Triggered Subsystem/Gripper Motor code generator  ==
  data: m1_cmd_low output; delta input; m1_cmd_high output; max_pos input; offset_grip input; prev_setpoint input; cur_setpoint output
function [m1_cmd_low, m1_cmd_high,cur_setpoint] =...
    code_gen_grip(delta,max_pos,offset_grip,prev_setpoint)

% New Control Effort
pos_setpoint =  prev_setpoint + delta;

% Check for Saturation
if (pos_setpoint >= max_pos)
	pos_setpoint = max_pos;
elseif (pos_setpoint <= 0)
    pos_setpoint = 0;
end
% Feedback setpoint for next time step
cur_setpoint = pos_setpoint;

% Add offset
motor_1_cmd  = uint16(abs(pos_setpoint)+offset_grip);

%% Prepare motor output
m1_cmd_low = uint8(uint16(192) + bitand(motor_1_cmd, uint16(31)));
m1_cmd_high = uint8(bitand(bitshift(motor_1_cmd, -5), uint16(127)));

end
